simulink library "EBCreator"  (R2018b)
settings: Solver=ode45  StartTime=0.0  StopTime=10.0  RelTol=1e-3  EnableMultiTasking=on
settings Model: Creator=lena.frank  LastModifiedBy=P41573
settings DataIOCC: LimitDataPoints=on  SaveFormat=Array  SignalLoggingSaveFormat=ModelDataLogs
settings OptimizationCC: ExpressionDepthLimit=2147483647  LifeSpan=inf
settings DebuggingCC: UnderspecifiedInitializationDetection=Classic  MergeDetectMultiDrivingBlocksExec=none  SolverPrmCheckMsg=warning  FcnCallInpInsideContextMsg=warning  StateNameClashWarn=warning  SFUnexpectedBacktrackingDiag=warning  SFNoUnconditionalDefaultTransitionDiag=warning  SFExecutionAtInitializationDiag=none
settings HardwareCC: ProdBitPerPointer=32  ProdBitPerSizeT=32  ProdBitPerPtrDiffT=32  ProdLargestAtomicFloat=None  ProdIntDivRoundTo=Undefined  ProdEndianess=Unspecified  ProdWordSize=32  ProdHWDeviceType=32-bit Generic
settings ModelReferenceCC: PropagateSignalLabelsOutOfModel=off
settings SFSimCC: SimUseLocalCustomCode=off
settings RTWCC: RTWUseLocalCustomCode=off
settings CodeAppCC: StateflowObjectComments=on
settings GRTTargetCC: TargetLangStandard=C89/C90 (ANSI)  GeneratePreprocessorConditionals=Disable all  CombineOutputUpdateFcns=off  GRTInterface=on
settings ConfigComp: CovMetricSettings=dw  CovHtmlReporting=on  CovSaveCumulativeToWorkspaceVar=on  CovSaveSingleToWorkspaceVar=on  CovExternalEMLEnable=off

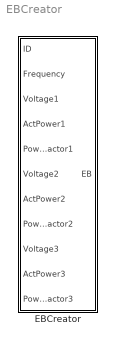
== system EBCreator ==
  EBCreator : Subsystem  InitFcn=load('EB.mat');  mask(EBCreator){Inport_ID=on, Inport_f=on, Inport_v1=on, Inport_p1=on, Inport_pf1=on, Inport_v2=on, Inport_p2=on, Inport_pf2=on, Inport_v3=on, Inport_p3=on, Inport_pf3=on, ID=4, f=50, v1=230, p1=0, pf1=1, v2=230, p2=0, pf2=1, v3=230, p3=0, pf3=1, Annotation_ID=off, Annotation_f=off, Annotation_v1=off, Annotation_p1=off, Annotation_pf1=off, Annotation_v2=off, Annotation_p2=off, Annotation_pf2=off, Annotation_v3=off, Annotation_p3=off, Annotation_pf3=on}
      mask prompts: Inport_ID "ID as inport"; Inport_f "frequency as inport"; Inport_v1 "voltage line 1 as inport"; Inport_p1 "active power line 1 as inport"; Inport_pf1 "power factor line 1 as inport"; Inport_v2 "voltage line 2 as inport"; Inport_p2 "active power line 1 as inport"; Inport_pf2 "power factor line 2 as inport"; Inport_v3 "voltage line 3 as inport"; Inport_p3 "active power line 3 as inport"; Inport_pf3 "power factor line 3 as inport"; ID "ID [1]"; f "frequency [Hz]"; v1 "voltage line 1 [V]"; p1 "active power line 1 [W]"; pf1 "power factor line 1 [1]"; v2 "voltage line 2 [V]"; p2 "active power line 2 [W]"; pf2 "power factor line 2 [1]"; v3 "voltage line 3 [V]"; p3 "active power line 3 [W]"; pf3 "power factor line 3 [1]"; Annotation_ID "ID as annotation"; Annotation_f "Frequency as annotation"; Annotation_v1 "voltage line 1 as annotation"; Annotation_p1 "active power line 1 as annotation"; Annotation_pf1 "fluid type as annotation"; Annotation_v2 "voltage line 2 as annotation"; Annotation_p2 "active power line 2 as annotation"; Annotation_pf2 "power factor line 2 as annotation"; Annotation_v3 "voltage line 3 as annotation"; Annotation_p3 "voltage line 3 as annotation"; Annotation_pf3 "power factor line 3 as annotation"
      mask help:
      | This block creates an EB from input signals.
      | ID is:
      | 1  Power only
      | 2  DC
      | 3  AC_1Phase
      | 4  AC_3Phase
      mask init:
      | CarnotCallbacks_EBCreator('CreateInports', gcb);
      mask Help: web(fullfile(path_carnot('help'),'EBCreator.html'),'-helpbrowser')
      mask Callback Inport_ID:
      | CarnotCallbacks_EBCreator('CreateMaskVisibilities', gcb);
      | CarnotCallbacks_EBCreator('CreateMaskAnnotations', gcb);
      mask Callback Inport_f:
      | CarnotCallbacks_EBCreator('CreateMaskVisibilities', gcb);
      | CarnotCallbacks_EBCreator('CreateMaskAnnotations', gcb);
      mask Callback Inport_v1:
      | CarnotCallbacks_EBCreator('CreateMaskVisibilities', gcb);
      | CarnotCallbacks_EBCreator('CreateMaskAnnotations', gcb);
      mask Callback Inport_p1:
      | CarnotCallbacks_EBCreator('CreateMaskVisibilities', gcb);
      | CarnotCallbacks_EBCreator('CreateMaskAnnotations', gcb);
      mask Callback Inport_pf1:
      | CarnotCallbacks_EBCreator('CreateMaskVisibilities', gcb);
      | CarnotCallbacks_EBCreator('CreateMaskAnnotations', gcb);
      mask Callback Inport_v2:
      | CarnotCallbacks_EBCreator('CreateMaskVisibilities', gcb);
      | CarnotCallbacks_EBCreator('CreateMaskAnnotations', gcb);
      mask Callback Inport_p2:
      | CarnotCallbacks_EBCreator('CreateMaskVisibilities', gcb);
      | CarnotCallbacks_EBCreator('CreateMaskAnnotations', gcb);
      mask Callback Inport_pf2:
      | CarnotCallbacks_EBCreator('CreateMaskVisibilities', gcb);
      | CarnotCallbacks_EBCreator('CreateMaskAnnotations', gcb);
      mask Callback Inport_v3:
      | CarnotCallbacks_EBCreator('CreateMaskVisibilities', gcb);
      | CarnotCallbacks_EBCreator('CreateMaskAnnotations', gcb);
      mask Callback Inport_p3:
      | CarnotCallbacks_EBCreator('CreateMaskVisibilities', gcb);
      | CarnotCallbacks_EBCreator('CreateMaskAnnotations', gcb);
      mask Callback Inport_pf3:
      | CarnotCallbacks_EBCreator('CreateMaskVisibilities', gcb);
      | CarnotCallbacks_EBCreator('CreateMaskAnnotations', gcb);
      mask Callback ID: CarnotCallbacks_EBCreator('CreateMaskAnnotations', gcb);
      mask Callback f: CarnotCallbacks_EBCreator('CreateMaskAnnotations', gcb);
      mask Callback v1: CarnotCallbacks_EBCreator('CreateMaskAnnotations', gcb);
      mask Callback p1: CarnotCallbacks_EBCreator('CreateMaskAnnotations', gcb);
      mask Callback pf1: CarnotCallbacks_EBCreator('CreateMaskAnnotations', gcb);
      mask Callback v2: CarnotCallbacks_EBCreator('CreateMaskAnnotations', gcb);
      mask Callback p2: CarnotCallbacks_EBCreator('CreateMaskAnnotations', gcb);
      mask Callback pf2: CarnotCallbacks_EBCreator('CreateMaskAnnotations', gcb);
      mask Callback v3: CarnotCallbacks_EBCreator('CreateMaskAnnotations', gcb);
      mask Callback p3: CarnotCallbacks_EBCreator('CreateMaskAnnotations', gcb);
      mask Callback pf3: CarnotCallbacks_EBCreator('CreateMaskAnnotations', gcb);
      mask Callback Annotation_ID: CarnotCallbacks_EBCreator('CreateMaskAnnotations', gcb);
      mask Callback Annotation_f: CarnotCallbacks_EBCreator('CreateMaskAnnotations', gcb);
      mask Callback Annotation_v1: CarnotCallbacks_EBCreator('CreateMaskAnnotations', gcb);
      mask Callback Annotation_p1: CarnotCallbacks_EBCreator('CreateMaskAnnotations', gcb);
      mask Callback Annotation_pf1: CarnotCallbacks_EBCreator('CreateMaskAnnotations', gcb);
      mask Callback Annotation_v2: CarnotCallbacks_EBCreator('CreateMaskAnnotations', gcb);
      mask Callback Annotation_p2: CarnotCallbacks_EBCreator('CreateMaskAnnotations', gcb);
      mask Callback Annotation_pf2: CarnotCallbacks_EBCreator('CreateMaskAnnotations', gcb);
      mask Callback Annotation_v3: CarnotCallbacks_EBCreator('CreateMaskAnnotations', gcb);
      mask Callback Annotation_p3: CarnotCallbacks_EBCreator('CreateMaskAnnotations', gcb);
      mask Callback Annotation_pf3: CarnotCallbacks_EBCreator('CreateMaskAnnotations', gcb);
      mask DialogControl ParameterTabVar0 Prompt: Settings
      mask DialogControl ParameterTabVar01 Prompt: Values
      mask DialogControl ParameterTabVar012 Prompt: Annotations

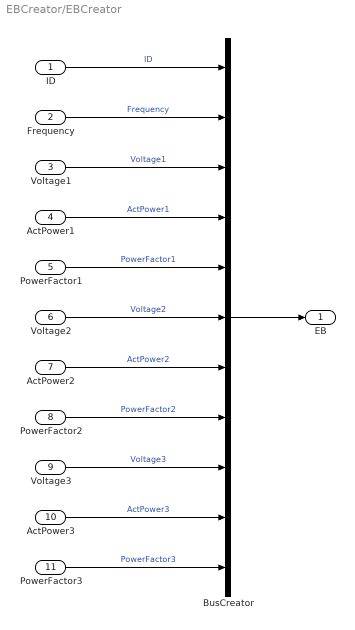
== system EBCreator/EBCreator ==
  ID : Inport
  Frequency : Inport  Port=2
  Voltage1 : Inport  Port=3
  ActPower1 : Inport  Port=4
  PowerFactor1 : Inport  Port=5
  Voltage2 : Inport  Port=6
  ActPower2 : Inport  Port=7
  PowerFactor2 : Inport  Port=8
  Voltage3 : Inport  Port=9
  ActPower3 : Inport  Port=10
  PowerFactor3 : Inport  Port=11
  BusCreator : BusCreator  Inputs=11  OutDataTypeStr=Bus: EB
      settings: InheritFromInputs=off
  EB : Outport  OutDataTypeStr=Bus: EB
  wires:
  BusCreator/1 -> EB/1
  ID/1 -> BusCreator/1  "ID"
  Frequency/1 -> BusCreator/2  "Frequency"
  Voltage1/1 -> BusCreator/3  "Voltage1"
  ActPower1/1 -> BusCreator/4  "ActPower1"
  PowerFactor1/1 -> BusCreator/5  "PowerFactor1"
  Voltage2/1 -> BusCreator/6  "Voltage2"
  ActPower2/1 -> BusCreator/7  "ActPower2"
  PowerFactor2/1 -> BusCreator/8  "PowerFactor2"
  Voltage3/1 -> BusCreator/9  "Voltage3"
  ActPower3/1 -> BusCreator/10  "ActPower3"
  PowerFactor3/1 -> BusCreator/11  "PowerFactor3"
